simulink model "A7E_requirements"  (R2012b)
settings: Solver=ode45  StartTime=0.0  StopTime=10.0  RelTol=1e-3
libraries: sldvlib x4
settings Model: Creator=roberto  LastModifiedBy=roberto

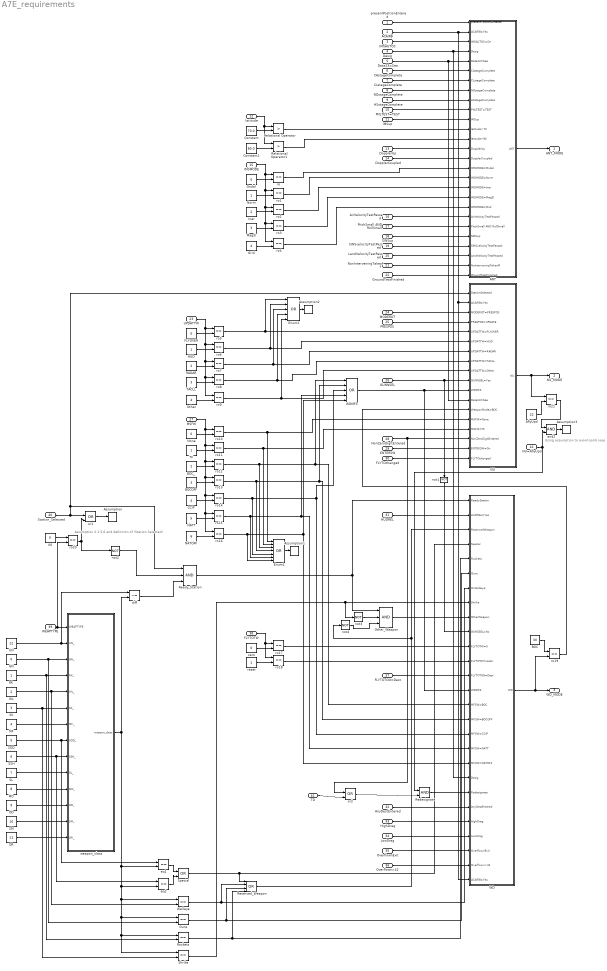
== system A7E_requirements ==
  note: Using assumption
      | to avoid comb loop
  note: Assumption 2.1.5.6
      | and definition
      | of !Station Selected!
  presentPositionEntered : Inport  OutDataTypeStr=boolean
  ACAIRB : Inport  Port=2  OutDataTypeStr=boolean
  IMSAUTOC : Inport  Port=3  OutDataTypeStr=boolean
  Desig : Inport  Port=4  OutDataTypeStr=boolean
  Data23=Sea : Inport  Port=5  OutDataTypeStr=boolean
  CAstageComplete : Inport  Port=6  OutDataTypeStr=boolean
  CLstageComplete : Inport  Port=7  OutDataTypeStr=boolean
  NDstageComplete : Inport  Port=8  OutDataTypeStr=boolean
  HSstageComplete : Inport  Port=9  OutDataTypeStr=boolean
  PNLTEST=TEST : Inport  Port=10  OutDataTypeStr=boolean
  IMSup : Inport  Port=11  OutDataTypeStr=boolean
  latitude : Inport  Port=12  OutDataTypeStr=double
  DopplerUp : Inport  Port=13  OutDataTypeStr=boolean
  DopplerCoupled : Inport  Port=14  OutDataTypeStr=boolean
  IMSMODE : Inport  Port=15  OutDataTypeStr=int8
  AirVelocityTestPassed : Inport  Port=16  OutDataTypeStr=boolean
  PitchSmall AND RollSmall : Inport  Port=17  OutDataTypeStr=boolean
  SINSup : Inport  Port=18  OutDataTypeStr=boolean
  SINSvelocityTestPassed : Inport  Port=19  OutDataTypeStr=boolean
  LandVelocityTestPassed : Inport  Port=20  OutDataTypeStr=boolean
  NonInterveningTakeoff : Inport  Port=21  OutDataTypeStr=boolean
  GroundTestFinished : Inport  Port=22  OutDataTypeStr=boolean
  UPDATTW : Inport  Port=23  OutDataTypeStr=int8
  MODEROT : Inport  Port=24  OutDataTypeStr=boolean
  PRESPOS : Inport  Port=25  OutDataTypeStr=boolean
  GUNNSEL : Inport  Port=26  OutDataTypeStr=boolean
  MSFW : Inport  Port=27  OutDataTypeStr=int8
  NonZeroDigitEntered : Inport  Port=28  OutDataTypeStr=boolean
  ENTERSW : Inport  Port=29  OutDataTypeStr=boolean
  FLYTOchanged : Inport  Port=30  OutDataTypeStr=boolean
  HUDREL : Inport  Port=31  OutDataTypeStr=boolean
  AnyDestEntered : Inport  Port=32  OutDataTypeStr=boolean
  HighDrag : Inport  Port=33  OutDataTypeStr=boolean
  LowDrag : Inport  Port=34  OutDataTypeStr=boolean
  OverflownExit : Inport  Port=35  OutDataTypeStr=boolean
  Overflown>42 : Inport  Port=36  OutDataTypeStr=boolean
  FLYTOTOG=Dest : Inport  Port=37  OutDataTypeStr=boolean
  FLYTOTW : Inport  Port=38  OutDataTypeStr=int8
  WEAPTYPE : Inport  Port=39  OutDataTypeStr=int8
  Station_Selected : Inport  Port=40  OutDataTypeStr=boolean
  TD : Inport  Port=41  OutDataTypeStr=boolean
  NU=AflyUpd : Inport  Port=42  OutDataTypeStr=boolean
  00 : Constant  Value=0  OutDataTypeStr=int8
  ANT : Subsystem
  AflyUpd : Constant  Value=22  OutDataTypeStr=int8
  Assumption{,1..3} (4 alike) : sldvlib/Objectives and Constraints/Assumption  enabled=on  customAVTBlockType=Assumption  intervals=true  initial=off  dispValues=on  outEnabled=on
      settings: AttributesFormatString=%<intervals>
  BOC : Constant  Value=30  OutDataTypeStr=int8
  BOCOFF : Constant  Value=3  OutDataTypeStr=int8
  BOC_ : Constant  Value=2  OutDataTypeStr=int8
  CCIP : Constant  Value=4  OutDataTypeStr=int8
  Constant : Constant  Value=70.0  OutDataTypeStr=double
  Constant1 : Constant  Value=80.0  OutDataTypeStr=double
  Enum1 : Logic  Operator=OR  Inputs=7  IconShape=distinctive  AllPortsSameDT=off  OutDataTypeStr=boolean
  Enum2 : Logic  Operator=OR  Inputs=5  IconShape=distinctive  AllPortsSameDT=off  OutDataTypeStr=boolean
  FLYOVER : Constant  Value=0  OutDataTypeStr=int8
  GN : Constant  Value=0  OutDataTypeStr=int8
  Gndal : Constant  Value=0  OutDataTypeStr=int8
  Grid : Constant  Value=4  OutDataTypeStr=int8
  Guns : RelationalOperator  Operator===  OutDataTypeStr=boolean
  HUD : Constant  OutDataTypeStr=int8
  Iner : Constant  Value=2  OutDataTypeStr=int8
  MD : Constant  Value=8  OutDataTypeStr=int8
  MF : Constant  Value=4  OutDataTypeStr=int8
  MagSl : Constant  Value=3  OutDataTypeStr=int8
  NATOFF : Constant  Value=6  OutDataTypeStr=int8
  NATT : Constant  Value=5  OutDataTypeStr=int8
  NU : Subsystem
  None : Constant  Value=0  OutDataTypeStr=int8
  Norm : Constant  OutDataTypeStr=int8
  OD : Constant  Value=9  OutDataTypeStr=int8
  OR : Constant  Value=11  OutDataTypeStr=int8
  Other : Constant  Value=4  OutDataTypeStr=int8
  Other_Weapon : Logic  Inputs=3  IconShape=distinctive  AllPortsSameDT=off  OutDataTypeStr=boolean
  RADAR : Constant  Value=2  OutDataTypeStr=int8
  RK : Constant  OutDataTypeStr=int8
  Ready_Station : Logic  Inputs=3  IconShape=distinctive  AllPortsSameDT=off  OutDataTypeStr=boolean
  Redesignate : Logic  IconShape=distinctive  AllPortsSameDT=off  OutDataTypeStr=boolean
  Relational Operator : RelationalOperator  Operator=>  OutDataTypeStr=boolean
  Relational Operator1 : RelationalOperator  Operator=>  OutDataTypeStr=boolean
  Reserved_Weapon : Logic  Operator=OR  Inputs=4  IconShape=distinctive  AllPortsSameDT=off  OutDataTypeStr=boolean
  Rockets : RelationalOperator  Operator===  OutDataTypeStr=boolean
  SK : Constant  Value=3  OutDataTypeStr=int8
  SL : Constant  Value=7  OutDataTypeStr=int8
  SM : Constant  Value=10  OutDataTypeStr=int8
  SOD : Constant  Value=5  OutDataTypeStr=int8
  SSH : Constant  Value=6  OutDataTypeStr=int8
  Shrike : RelationalOperator  Operator===  OutDataTypeStr=boolean
  Special : Logic  Operator=OR  IconShape=distinctive  AllPortsSameDT=off  OutDataTypeStr=boolean
  TACLL : Constant  Value=3  OutDataTypeStr=int8
  TF : Constant  OutDataTypeStr=int8
  UN : Constant  Value=12  OutDataTypeStr=int8
  WD : Subsystem
  WDMFS : Logic  Operator=OR  Inputs=5  IconShape=distinctive  AllPortsSameDT=off  OutDataTypeStr=boolean
  WL : Constant  Value=2  OutDataTypeStr=int8
  Walleye : RelationalOperator  Operator===  OutDataTypeStr=boolean
  and2 : Logic  IconShape=distinctive  AllPortsSameDT=off  OutDataTypeStr=boolean
  diff : RelationalOperator  Operator=~=  OutDataTypeStr=boolean
  eq1 : RelationalOperator  Operator===  OutDataTypeStr=boolean
  eq2 : RelationalOperator  Operator===  OutDataTypeStr=boolean
  not1 : Logic  Operator=NOT  IconShape=distinctive  AllPortsSameDT=off  OutDataTypeStr=boolean
  not2 : Logic  Operator=NOT  Inputs=3  IconShape=distinctive  AllPortsSameDT=off  OutDataTypeStr=boolean
  not3 : Logic  Operator=NOT  Inputs=3  IconShape=distinctive  AllPortsSameDT=off  OutDataTypeStr=boolean
  not4 : Logic  Operator=NOT  Inputs=3  IconShape=distinctive  AllPortsSameDT=off  OutDataTypeStr=boolean
  or1 : Logic  Operator=OR  IconShape=distinctive  AllPortsSameDT=off  OutDataTypeStr=boolean
  or2 : Logic  Operator=OR  IconShape=distinctive  AllPortsSameDT=off  OutDataTypeStr=boolean
  reset : Constant  OutDataTypeStr=int8
  ro{,1..21} (22 alike) : RelationalOperator  Operator===  OutDataTypeStr=boolean
  weapon_class : Subsystem
  zero : Constant  Value=0  OutDataTypeStr=int8
  ANT_MODE : Outport
  NU_MODE : Outport  Port=2
  WD_MODE : Outport  Port=3
  wires:
  presentPositionEntered/1 -> ANT/1(presentPositionEntered)
  ACAIRB/1 -> WD/27(ACAIRB=Yes), NU/2(ACAIRB=Yes), ANT/2(ACAIRB=Yes)
  IMSAUTOC/1 -> ANT/3(IMSAUTOC=On)
  Desig/1 -> WD/20(Desig), ANT/4(Desig)
  Data23=Sea/1 -> NU/12(Data23=Sea), ANT/5(Data23=Sea)
  CAstageComplete/1 -> ANT/6(CAstageComplete)
  CLstageComplete/1 -> ANT/7(CLstageComplete)
  NDstageComplete/1 -> ANT/8(NDstageComplete)
  HSstageComplete/1 -> ANT/9(HSstageComplete)
  PNLTEST=TEST/1 -> ANT/10(PNLTEST=TEST)
  IMSup/1 -> ANT/11(IMSup)
  DopplerUp/1 -> ANT/14(DopplerUp)
  DopplerCoupled/1 -> ANT/15(DopplerCoupled)
  AirVelocityTestPassed/1 -> ANT/21(AirVelocityTestPassed)
  PitchSmall AND RollSmall/1 -> ANT/22(PitchSmall AND RollSmall)
  ANT/1(ANT) -> ANT_MODE/1
  Station_Selected/1 -> NU/1(StationSelected), Ready_Station/1, or1/1
  latitude/1 -> Relational Operator1/1, Relational Operator/1
  Constant/1 -> Relational Operator/2
  Constant1/1 -> Relational Operator1/2
  Relational Operator1/1 -> ANT/13(latitude>80)
  Relational Operator/1 -> ANT/12(latitude>70)
  IMSMODE/1 -> ro/1, ro4/1, ro3/1, ro2/1, ro1/1
  Gndal/1 -> ro/2
  Norm/1 -> ro1/2
  Iner/1 -> ro2/2
  MagSl/1 -> ro3/2
  Grid/1 -> ro4/2
  ro/1 -> ANT/16(IMSMODE=Gndal)
  ro1/1 -> ANT/17(IMSMODE=Norm)
  ro2/1 -> ANT/18(IMSMODE=Iner)
  ro3/1 -> ANT/19(IMSMODE=MagSl)
  ro4/1 -> ANT/20(IMSMODE=Grid)
  UPDATTW/1 -> ro5/1, ro9/1, ro8/1, ro7/1, ro6/1
  FLYOVER/1 -> ro5/2
  HUD/1 -> ro6/2
  RADAR/1 -> ro7/2
  TACLL/1 -> ro8/2
  Other/1 -> ro9/2
  ro5/1 -> Enum2/1, NU/5(UPDATTW=FLYOVER)
  ro6/1 -> Enum2/2, NU/6(UPDATTW=HUD)
  ro7/1 -> Enum2/3, NU/7(UPDATTW=RADAR)
  ro8/1 -> Enum2/4, NU/8(UPDATTW=TACLL)
  ro9/1 -> Enum2/5, NU/9(UPDATTW=Other)
  MODEROT/1 -> NU/3(MODEROT=PRESPOS)
  PRESPOS/1 -> NU/4(PRESPOS=UPDATE)
  GUNNSEL/1 -> not1/1, NU/10(GUNNSEL=Yes)
  MSFW/1 -> ro10/1, ro16/1, ro15/1, ro14/1, ro13/1, ro12/1, ro11/1
  None/1 -> ro10/2
  TF/1 -> ro11/2
  BOC_/1 -> ro12/2
  BOCOFF/1 -> ro13/2
  CCIP/1 -> ro14/2
  NATT/1 -> ro15/2
  NATOFF/1 -> ro16/2
  ro10/1 -> Enum1/1, NU/14(MSFW=None)
  ro11/1 -> Enum1/2, NU/15(MSFW=TF)
  ro12/1 -> Enum1/3, WDMFS/1, WD/15(MFSW=BOC)
  ro13/1 -> Enum1/4, WDMFS/2, WD/16(MFSW=BOCOFF)
  ro14/1 -> Enum1/5, WD/17(MFSW=CCIP), WDMFS/3
  ro16/1 -> Enum1/7, WD/19(MFSW=NATOFF), WDMFS/5
  NonZeroDigitEntered/1 -> or2/1, NU/16(NonZeroDigitEntered)
  ENTERSW/1 -> NU/17(ENTERSW=On)
  FLYTOchanged/1 -> NU/18(FLYTOchanged)
  Ready_Station/1 -> WD/1(ReadyStation), Other_Weapon/1
  HUDREL/1 -> WD/2(HUDREL=Yes)
  Special/1 -> Reserved_Weapon/1, WD/4(Special)
  Walleye/1 -> Reserved_Weapon/2, WD/7(OnWalleye)
  Other_Weapon/1 -> WD/9(OtherWeapon)
  not1/1 -> WD/10(GUNSSEL=No)
  WDMFS/1 -> WD/14(WDMFS), NU/11(WDMFS)
  AnyDestEntered/1 -> WD/22(AnyDestEntered)
  HighDrag/1 -> WD/23(HighDrag)
  LowDrag/1 -> WD/24(LowDrag)
  OverflownExit/1 -> WD/25(OverflownExit)
  Overflown>42/1 -> WD/26(Overflown>42)
  FLYTOTOG=Dest/1 -> WD/13(FLYTOTOG=Dest)
  FLYTOTW/1 -> ro17/1, ro18/1
  zero/1 -> ro17/2
  reset/1 -> ro18/2
  ro17/1 -> WD/11(FLYTOTW=0)
  ro18/1 -> WD/12(FLYTOTW=reset)
  GroundTestFinished/1 -> ANT/27(GroundTestFinished)
  NonInterveningTakeoff/1 -> ANT/26(NoInterveningTakeoff)
  SINSup/1 -> ANT/23(SINSup)
  SINSvelocityTestPassed/1 -> ANT/24(SINSvelocityTestPassed)
  LandVelocityTestPassed/1 -> ANT/25(LandVelocityTestPassed)
  NU/1(NU) -> ro21/1, NU_MODE/1
  WD/1(WD) -> ro19/2, WD_MODE/1
  BOC/1 -> ro19/1
  ro19/1 -> NU/13(WeaponMode=BOC)
  WEAPTYPE/1 -> weapon_class/1(WEAPTYPE), ro20/2
  UN/1 -> diff/1, weapon_class/2(UN_)
  GN/1 -> Guns/2, weapon_class/3(GN_)
  RK/1 -> Rockets/2, weapon_class/4(RK_)
  SK/1 -> Shrike/2, weapon_class/6(SK_)
  MF/1 -> weapon_class/7(MF_)
  SOD/1 -> eq1/1, weapon_class/8(SOD_)
  SSH/1 -> eq2/1, weapon_class/9(SSH_)
  SL/1 -> weapon_class/10(SL_)
  MD/1 -> weapon_class/11(MD_)
  OD/1 -> weapon_class/12(OD_)
  SM/1 -> weapon_class/13(SM_)
  OR/1 -> weapon_class/14(OR_)
  00/1 -> ro20/1
  ro20/1 -> or1/2, not2/1
  or1/1 -> Assumption/1
  not2/1 -> Ready_Station/2
  diff/1 -> Ready_Station/3
  weapon_class/1(weapon_class) -> diff/2, Shrike/1, Rockets/1, Guns/1, Walleye/1, eq2/2, eq1/2
  eq1/1 -> Special/1
  eq2/1 -> Special/2
  WL/1 -> Walleye/2, weapon_class/5(WL_)
  Guns/1 -> Reserved_Weapon/3, WD/6(Guns)
  Rockets/1 -> Reserved_Weapon/4, WD/5(Rockets)
  Shrike/1 -> not3/1, WD/8(Shrike)
  Reserved_Weapon/1 -> WD/3(ReservedWeapon), not4/1
  not3/1 -> Other_Weapon/2
  not4/1 -> Other_Weapon/3
  ro15/1 -> Enum1/6, WDMFS/4, WD/18(MFSW=NATT)
  Enum1/1 -> Assumption1/1
  Enum2/1 -> Assumption2/1
  TD/1 -> or2/2
  or2/1 -> Redesignate/2
  Redesignate/1 -> WD/21(Redesignate)
  AflyUpd/1 -> ro21/2
  NU=AflyUpd/1 -> Redesignate/1, and2/2
  ro21/1 -> and2/1
  and2/1 -> Assumption3/1

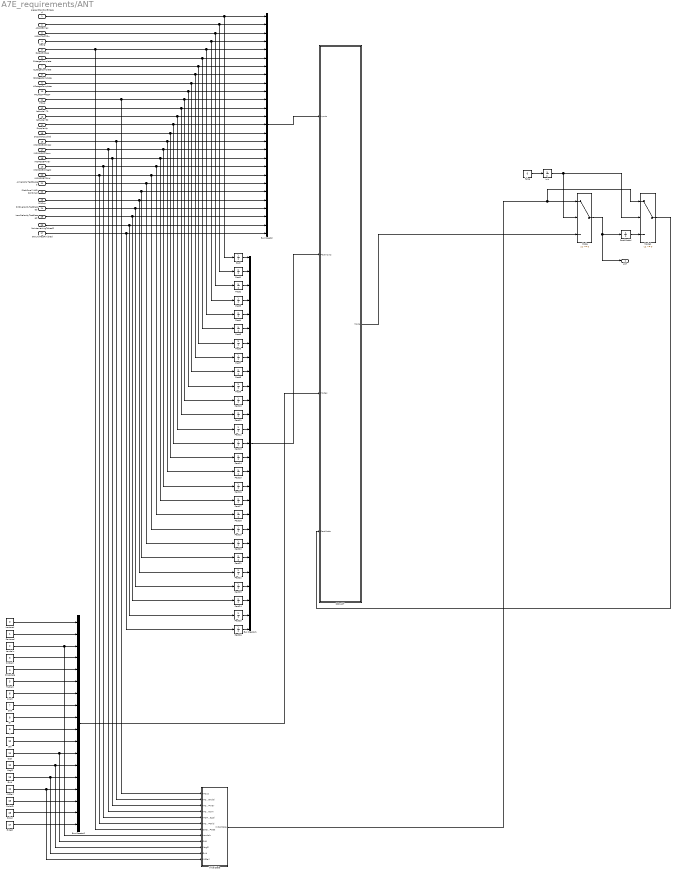
== system A7E_requirements/ANT ==
  presentPositionEntered : Inport  OutDataTypeStr=boolean
  ACAIRB=Yes : Inport  Port=2  OutDataTypeStr=boolean
  IMSAUTOC=On : Inport  Port=3  OutDataTypeStr=boolean
  Desig : Inport  Port=4  OutDataTypeStr=boolean
  Data23=Sea : Inport  Port=5  OutDataTypeStr=boolean
  CAstageComplete : Inport  Port=6  OutDataTypeStr=boolean
  CLstageComplete : Inport  Port=7  OutDataTypeStr=boolean
  NDstageComplete : Inport  Port=8  OutDataTypeStr=boolean
  HSstageComplete : Inport  Port=9  OutDataTypeStr=boolean
  PNLTEST=TEST : Inport  Port=10  OutDataTypeStr=boolean
  IMSup : Inport  Port=11  OutDataTypeStr=boolean
  latitude>70 : Inport  Port=12  OutDataTypeStr=boolean
  latitude>80 : Inport  Port=13  OutDataTypeStr=boolean
  DopplerUp : Inport  Port=14  OutDataTypeStr=boolean
  DopplerCoupled : Inport  Port=15  OutDataTypeStr=boolean
  IMSMODE=Gndal : Inport  Port=16  OutDataTypeStr=boolean
  IMSMODE=Norm : Inport  Port=17  OutDataTypeStr=boolean
  IMSMODE=Iner : Inport  Port=18  OutDataTypeStr=boolean
  IMSMODE=MagSl : Inport  Port=19  OutDataTypeStr=boolean
  IMSMODE=Grid : Inport  Port=20  OutDataTypeStr=boolean
  AirVelocityTestPassed : Inport  Port=21  OutDataTypeStr=boolean
  PitchSmall AND RollSmall : Inport  Port=22  OutDataTypeStr=boolean
  SINSup : Inport  Port=23  OutDataTypeStr=boolean
  SINSvelocityTestPassed : Inport  Port=24  OutDataTypeStr=boolean
  LandVelocityTestPassed : Inport  Port=25  OutDataTypeStr=boolean
  NoInterveningTakeoff : Inport  Port=26  OutDataTypeStr=boolean
  GroundTestFinished : Inport  Port=27  OutDataTypeStr=boolean
  01Update : Constant  Value=4  OutDataTypeStr=int8
  Airaln : Constant  Value=6  OutDataTypeStr=int8
  Bus Creator : BusCreator  Inputs=27
  Bus Creator1 : BusCreator  Inputs=27
  Bus Creator2 : BusCreator  Inputs=18
  DI : Constant  Value=8  OutDataTypeStr=int8
  DIG : Constant  Value=7  OutDataTypeStr=int8
  Grid : Constant  Value=13  OutDataTypeStr=int8
  Grtest : Constant  Value=17  OutDataTypeStr=int8
  HUDaln : Constant  Value=5  OutDataTypeStr=int8
  I : Constant  Value=9  OutDataTypeStr=int8
  IMSfail : Constant  Value=14  OutDataTypeStr=int8
  Init : UnitDelay  InitialCondition=1  SampleTime=-1
  InitialState : Subsystem
  Landaln : Constant  Value=2  OutDataTypeStr=int8
  Lautocal : Constant  Value=0  OutDataTypeStr=int8
  MagSl : Constant  Value=12  OutDataTypeStr=int8
  Mode : Switch  Criteria=u2 ~= 0  OutDataTypeStr=int8
  Mode1 : Switch  Criteria=u2 ~= 0  OutDataTypeStr=int8
  OLB : Constant  Value=11  OutDataTypeStr=int8
  Past{,1..26} (27 alike) : UnitDelay  InitialCondition=1  SampleTime=-1
  Past(Mode) : UnitDelay  InitialCondition=1  SampleTime=-1
  PolarDI : Constant  Value=15  OutDataTypeStr=int8
  PolarI : Constant  Value=16  OutDataTypeStr=int8
  SCR:ANT : Subsystem
  SINSaln : Constant  Value=3  OutDataTypeStr=int8
  Sautocal : Constant  OutDataTypeStr=int8
  UDI : Constant  Value=10  OutDataTypeStr=int8
  false : Constant  Value=0  OutDataTypeStr=boolean
  ANT : Outport
  wires:
  Past1/1 -> Bus Creator1/2
  Past4/1 -> Bus Creator1/5
  Past23/1 -> Bus Creator1/24
  Past20/1 -> Bus Creator1/21
  Past21/1 -> Bus Creator1/22
  Past6/1 -> Bus Creator1/7
  Past22/1 -> Bus Creator1/23
  Past5/1 -> Bus Creator1/6
  Past7/1 -> Bus Creator1/8
  Past24/1 -> Bus Creator1/25
  Past3/1 -> Bus Creator1/4
  Past2/1 -> Bus Creator1/3
  Past8/1 -> Bus Creator1/9
  Past9/1 -> Bus Creator1/10
  Past12/1 -> Bus Creator1/13
  Past11/1 -> Bus Creator1/12
  Past10/1 -> Bus Creator1/11
  Past17/1 -> Bus Creator1/18
  Past13/1 -> Bus Creator1/14
  Past14/1 -> Bus Creator1/15
  Past15/1 -> Bus Creator1/16
  Past18/1 -> Bus Creator1/19
  Past16/1 -> Bus Creator1/17
  Past19/1 -> Bus Creator1/20
  CLstageComplete/1 -> Past6/1, Bus Creator/7
  CAstageComplete/1 -> Past5/1, Bus Creator/6
  NDstageComplete/1 -> Past7/1, Bus Creator/8
  OLB/1 -> InitialState/9(OLB), Bus Creator2/12
  01Update/1 -> Bus Creator2/5
  HUDaln/1 -> Bus Creator2/6
  Airaln/1 -> Bus Creator2/7
  IMSfail/1 -> InitialState/12(IMSfail), Bus Creator2/15
  presentPositionEntered/1 -> Past/1, Bus Creator/1
  ACAIRB=Yes/1 -> Past1/1, Bus Creator/2
  PitchSmall AND RollSmall/1 -> Past21/1, Bus Creator/22
  SINSup/1 -> Past22/1, Bus Creator/23
  DopplerCoupled/1 -> Past14/1, Bus Creator/15
  PNLTEST=TEST/1 -> Past9/1, Bus Creator/10
  IMSMODE=Iner/1 -> InitialState/3(IMSMODE=Iner), Past17/1, Bus Creator/18
  IMSMODE=MagSl/1 -> InitialState/5(IMSMODE=MagSl), Past18/1, Bus Creator/19
  LandVelocityTestPassed/1 -> Past24/1, Bus Creator/25
  SINSvelocityTestPassed/1 -> Past23/1, Bus Creator/24
  latitude>80/1 -> Past12/1, Bus Creator/13
  IMSup/1 -> InitialState/1(IMSup), Past10/1, Bus Creator/11
  IMSMODE=Norm/1 -> InitialState/4(IMSMODE=Norm), Past16/1, Bus Creator/17
  AirVelocityTestPassed/1 -> Past20/1, Bus Creator/21
  IMSMODE=Grid/1 -> InitialState/6(IMSMODE=Grid), Past19/1, Bus Creator/20
  DopplerUp/1 -> Past13/1, Bus Creator/14
  HSstageComplete/1 -> Past8/1, Bus Creator/9
  IMSMODE=Gndal/1 -> InitialState/2(IMSMODE=Gndal), Past15/1, Bus Creator/16
  latitude>70/1 -> Past11/1, Bus Creator/12
  IMSAUTOC=On/1 -> Past2/1, Bus Creator/3
  Desig/1 -> Past3/1, Bus Creator/4
  Sautocal/1 -> Bus Creator2/2
  Landaln/1 -> Bus Creator2/3, InitialState/8(Landaln)
  SINSaln/1 -> Bus Creator2/4
  Past/1 -> Bus Creator1/1
  Mode/1 -> Past(Mode)/1, ANT/1
  Mode1/1 -> SCR:ANT/4(PastMode)
  SCR:ANT/1(Mode) -> Mode/3
  Bus Creator2/1 -> SCR:ANT/3(Modes)
  Bus Creator/1 -> SCR:ANT/1(Inputs)
  Bus Creator1/1 -> SCR:ANT/2(PastInputs)
  Init/1 -> Mode/2, Mode1/2
  Lautocal/1 -> Bus Creator2/1
  false/1 -> Init/1
  DI/1 -> Bus Creator2/9
  I/1 -> Bus Creator2/10
  DIG/1 -> Bus Creator2/8
  Grid/1 -> InitialState/11(Grid), Bus Creator2/14
  Grtest/1 -> Bus Creator2/18
  PolarI/1 -> Bus Creator2/17
  PolarDI/1 -> Bus Creator2/16
  UDI/1 -> Bus Creator2/11
  InitialState/1(InitialState) -> Mode1/1, Mode/1
  MagSl/1 -> InitialState/10(MagSl), Bus Creator2/13
  Data23=Sea/1 -> InitialState/7(Data23=Sea), Past4/1, Bus Creator/5
  NoInterveningTakeoff/1 -> Past25/1, Bus Creator/26
  GroundTestFinished/1 -> Past26/1, Bus Creator/27
  Past25/1 -> Bus Creator1/26
  Past26/1 -> Bus Creator1/27
  Past(Mode)/1 -> Mode1/3

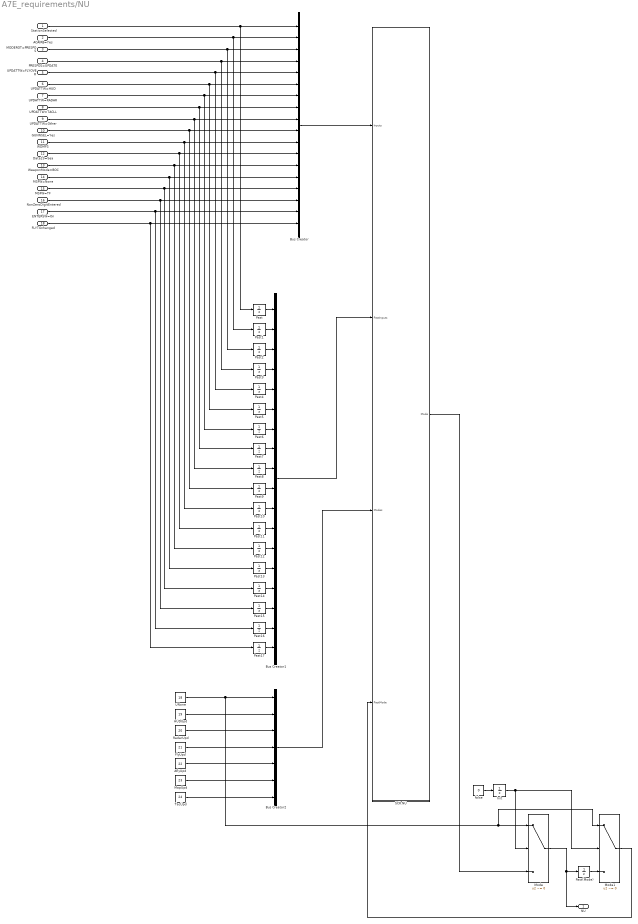
== system A7E_requirements/NU ==
  StationSelected : Inport  OutDataTypeStr=boolean
  ACAIRB=Yes : Inport  Port=2  OutDataTypeStr=boolean
  MODEROT=PRESPOS : Inport  Port=3  OutDataTypeStr=boolean
  PRESPOS=UPDATE : Inport  Port=4  OutDataTypeStr=boolean
  UPDATTW=FLYOVER : Inport  Port=5  OutDataTypeStr=boolean
  UPDATTW=HUD : Inport  Port=6  OutDataTypeStr=boolean
  UPDATTW=RADAR : Inport  Port=7  OutDataTypeStr=boolean
  UPDATTW=TACLL : Inport  Port=8  OutDataTypeStr=boolean
  UPDATTW=Other : Inport  Port=9  OutDataTypeStr=boolean
  GUNNSEL=Yes : Inport  Port=10  OutDataTypeStr=boolean
  WDMFS : Inport  Port=11  OutDataTypeStr=boolean
  Data23=Sea : Inport  Port=12  OutDataTypeStr=boolean
  WeaponMode=BOC : Inport  Port=13  OutDataTypeStr=boolean
  MSFW=None : Inport  Port=14  OutDataTypeStr=boolean
  MSFW=TF : Inport  Port=15  OutDataTypeStr=boolean
  NonZeroDigitEntered : Inport  Port=16  OutDataTypeStr=boolean
  ENTERSW=On : Inport  Port=17  OutDataTypeStr=boolean
  FLYTOchanged : Inport  Port=18  OutDataTypeStr=boolean
  AflyUpd : Constant  Value=22  OutDataTypeStr=int8
  Bus Creator : BusCreator  Inputs=18
  Bus Creator1 : BusCreator  Inputs=18
  Bus Creator2 : BusCreator  Inputs=7
  FlyUpd : Constant  Value=21  OutDataTypeStr=int8
  HUDUpd : Constant  Value=19  OutDataTypeStr=int8
  Init : UnitDelay  InitialCondition=1  SampleTime=-1
  MapUpd : Constant  Value=23  OutDataTypeStr=int8
  Mode : Switch  Criteria=u2 ~= 0
  Mode1 : Switch  Criteria=u2 ~= 0
  Past{,1..17} (18 alike) : UnitDelay  InitialCondition=1  SampleTime=-1
  Past(Mode) : UnitDelay  InitialCondition=1  SampleTime=-1
  RadarUpd : Constant  Value=20  OutDataTypeStr=int8
  SCR:NU : Subsystem
  TacUpd : Constant  Value=24  OutDataTypeStr=int8
  UNone : Constant  Value=18  OutDataTypeStr=int8
  false : Constant  Value=0  OutDataTypeStr=boolean
  NU : Outport  OutDataTypeStr=int8
  wires:
  Past1/1 -> Bus Creator1/2
  Past4/1 -> Bus Creator1/5
  Past6/1 -> Bus Creator1/7
  Past5/1 -> Bus Creator1/6
  Past7/1 -> Bus Creator1/8
  Past3/1 -> Bus Creator1/4
  Past2/1 -> Bus Creator1/3
  Past8/1 -> Bus Creator1/9
  Past9/1 -> Bus Creator1/10
  Past12/1 -> Bus Creator1/13
  Past11/1 -> Bus Creator1/12
  Past10/1 -> Bus Creator1/11
  Past17/1 -> Bus Creator1/18
  Past13/1 -> Bus Creator1/14
  Past14/1 -> Bus Creator1/15
  Past15/1 -> Bus Creator1/16
  Past16/1 -> Bus Creator1/17
  UPDATTW=RADAR/1 -> Past6/1, Bus Creator/7
  UPDATTW=HUD/1 -> Past5/1, Bus Creator/6
  UPDATTW=TACLL/1 -> Past7/1, Bus Creator/8
  UPDATTW=FLYOVER/1 -> Past4/1, Bus Creator/5
  StationSelected/1 -> Past/1, Bus Creator/1
  ACAIRB=Yes/1 -> Past1/1, Bus Creator/2
  MSFW=TF/1 -> Past14/1, Bus Creator/15
  GUNNSEL=Yes/1 -> Past9/1, Bus Creator/10
  FLYTOchanged/1 -> Past17/1, Bus Creator/18
  WeaponMode=BOC/1 -> Past12/1, Bus Creator/13
  WDMFS/1 -> Past10/1, Bus Creator/11
  ENTERSW=On/1 -> Past16/1, Bus Creator/17
  MSFW=None/1 -> Past13/1, Bus Creator/14
  UPDATTW=Other/1 -> Past8/1, Bus Creator/9
  NonZeroDigitEntered/1 -> Past15/1, Bus Creator/16
  Data23=Sea/1 -> Past11/1, Bus Creator/12
  MODEROT=PRESPOS/1 -> Past2/1, Bus Creator/3
  PRESPOS=UPDATE/1 -> Past3/1, Bus Creator/4
  Past/1 -> Bus Creator1/1
  Mode/1 -> Past(Mode)/1, NU/1
  Mode1/1 -> SCR:NU/4(PastMode)
  SCR:NU/1(Mode) -> Mode/3
  Bus Creator2/1 -> SCR:NU/3(Modes)
  Bus Creator/1 -> SCR:NU/1(Inputs)
  Bus Creator1/1 -> SCR:NU/2(PastInputs)
  Init/1 -> Mode/2, Mode1/2
  false/1 -> Init/1
  UNone/1 -> Mode1/1, Mode/1, Bus Creator2/1
  HUDUpd/1 -> Bus Creator2/2
  RadarUpd/1 -> Bus Creator2/3
  FlyUpd/1 -> Bus Creator2/4
  AflyUpd/1 -> Bus Creator2/5
  MapUpd/1 -> Bus Creator2/6
  TacUpd/1 -> Bus Creator2/7
  Past(Mode)/1 -> Mode1/3

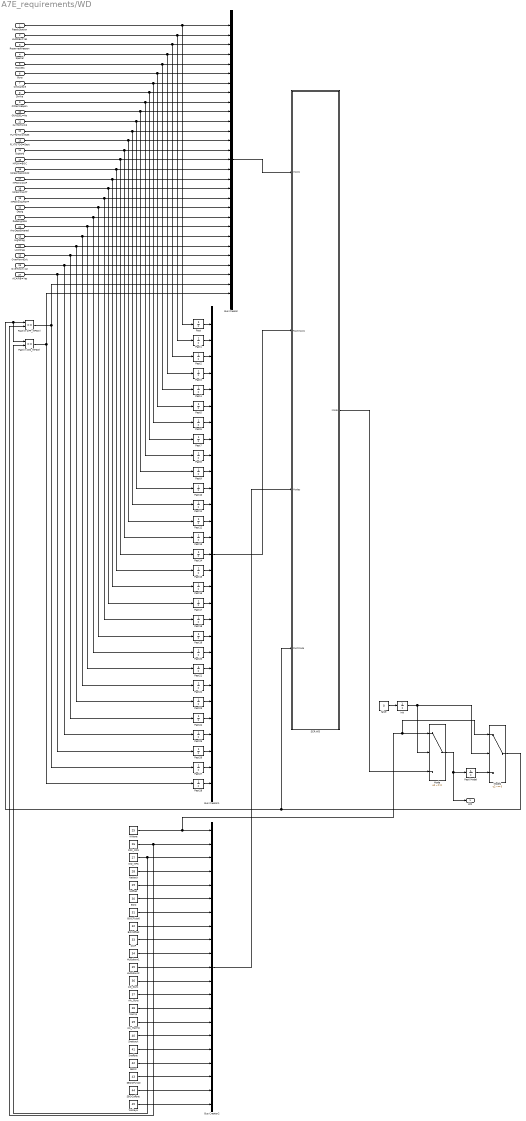
== system A7E_requirements/WD ==
  ReadyStation : Inport  OutDataTypeStr=boolean
  HUDREL=Yes : Inport  Port=2  OutDataTypeStr=boolean
  ReservedWeapon : Inport  Port=3  OutDataTypeStr=boolean
  Special : Inport  Port=4  OutDataTypeStr=boolean
  Rockets : Inport  Port=5  OutDataTypeStr=boolean
  Guns : Inport  Port=6  OutDataTypeStr=boolean
  OnWalleye : Inport  Port=7  OutDataTypeStr=boolean
  Shrike : Inport  Port=8  OutDataTypeStr=boolean
  OtherWeapon : Inport  Port=9  OutDataTypeStr=boolean
  GUNSSEL=No : Inport  Port=10  OutDataTypeStr=boolean
  FLYTOTW=0 : Inport  Port=11  OutDataTypeStr=boolean
  FLYTOTW=reset : Inport  Port=12  OutDataTypeStr=boolean
  FLYTOTOG=Dest : Inport  Port=13  OutDataTypeStr=boolean
  WDMFS : Inport  Port=14  OutDataTypeStr=boolean
  MFSW=BOC : Inport  Port=15  OutDataTypeStr=boolean
  MFSW=BOCOFF : Inport  Port=16  OutDataTypeStr=boolean
  MFSW=CCIP : Inport  Port=17  OutDataTypeStr=boolean
  MFSW=NATT : Inport  Port=18  OutDataTypeStr=boolean
  MFSW=NATOFF : Inport  Port=19  OutDataTypeStr=boolean
  Desig : Inport  Port=20  OutDataTypeStr=boolean
  Redesignate : Inport  Port=21  OutDataTypeStr=boolean
  AnyDestEntered : Inport  Port=22  OutDataTypeStr=boolean
  HighDrag : Inport  Port=23  OutDataTypeStr=boolean
  LowDrag : Inport  Port=24  OutDataTypeStr=boolean
  OverflownExit : Inport  Port=25  OutDataTypeStr=boolean
  Overflown>42 : Inport  Port=26  OutDataTypeStr=boolean
  ACAIRB=Yes : Inport  Port=27  OutDataTypeStr=boolean
  AA_Guns : Constant  Value=37  OutDataTypeStr=int8
  AA_Manrip : Constant  Value=39  OutDataTypeStr=int8
  AG_Guns : Constant  Value=36  OutDataTypeStr=int8
  BOC : Constant  Value=30  OutDataTypeStr=int8
  BOCFlyto0 : Constant  Value=31  OutDataTypeStr=int8
  BOCoffset : Constant  Value=32  OutDataTypeStr=int8
  Bus Creator : BusCreator  Inputs=29
  Bus Creator1 : BusCreator  Inputs=29
  Bus Creator2 : BusCreator  Inputs=21
  CCIP : Constant  Value=33  OutDataTypeStr=int8
  HUDdown1 : Constant  Value=34  OutDataTypeStr=int8
  HUDdown2 : Constant  Value=35  OutDataTypeStr=int8
  Init : UnitDelay  InitialCondition=1  SampleTime=-1
  Manrip : Constant  Value=38  OutDataTypeStr=int8
  Mode : Switch  Criteria=u2 ~= 0
  Mode1 : Switch  Criteria=u2 ~= 0
  Nattack : Constant  Value=28  OutDataTypeStr=int8
  Noffset : Constant  Value=29  OutDataTypeStr=int8
  OFF_MFS : Constant  Value=26  OutDataTypeStr=int8
  Past{,1..28} (29 alike) : UnitDelay  InitialCondition=1  SampleTime=-1
  Past(In OFF_MFSW) : RelationalOperator  Operator===  OutDataTypeStr=boolean
  Past(In WD_MFSW) : RelationalOperator  Operator===  OutDataTypeStr=boolean
  Past(Mode) : UnitDelay  InitialCondition=1  SampleTime=-1
  SBOC : Constant  Value=42  OutDataTypeStr=int8
  SBOCFlyto0 : Constant  Value=43  OutDataTypeStr=int8
  SBOCoffset : Constant  Value=44  OutDataTypeStr=int8
  SCR:WD : Subsystem
  Snattack : Constant  Value=40  OutDataTypeStr=int8
  Snoffset : Constant  Value=41  OutDataTypeStr=int8
  WD_MFS : Constant  Value=27  OutDataTypeStr=int8
  WNone : Constant  Value=25  OutDataTypeStr=int8
  Walleye : Constant  Value=45  OutDataTypeStr=int8
  false : Constant  Value=0  OutDataTypeStr=boolean
  WD : Outport
  wires:
  Past1/1 -> Bus Creator1/2
  Past4/1 -> Bus Creator1/5
  Past23/1 -> Bus Creator1/24
  Past20/1 -> Bus Creator1/21
  Past21/1 -> Bus Creator1/22
  Past6/1 -> Bus Creator1/7
  Past22/1 -> Bus Creator1/23
  Past5/1 -> Bus Creator1/6
  Past7/1 -> Bus Creator1/8
  Past24/1 -> Bus Creator1/25
  Past3/1 -> Bus Creator1/4
  Past2/1 -> Bus Creator1/3
  Past8/1 -> Bus Creator1/9
  Past9/1 -> Bus Creator1/10
  Past12/1 -> Bus Creator1/13
  Past11/1 -> Bus Creator1/12
  Past10/1 -> Bus Creator1/11
  Past17/1 -> Bus Creator1/18
  Past13/1 -> Bus Creator1/14
  Past14/1 -> Bus Creator1/15
  Past15/1 -> Bus Creator1/16
  Past18/1 -> Bus Creator1/19
  Past16/1 -> Bus Creator1/17
  Past19/1 -> Bus Creator1/20
  OnWalleye/1 -> Past6/1, Bus Creator/7
  Guns/1 -> Past5/1, Bus Creator/6
  Shrike/1 -> Past7/1, Bus Creator/8
  Rockets/1 -> Past4/1, Bus Creator/5
  AG_Guns/1 -> Bus Creator2/12
  BOC/1 -> Bus Creator2/6
  BOCFlyto0/1 -> Bus Creator2/7
  AA_Manrip/1 -> Bus Creator2/15
  ReadyStation/1 -> Past/1, Bus Creator/1
  HUDREL=Yes/1 -> Past1/1, Bus Creator/2
  AnyDestEntered/1 -> Past21/1, Bus Creator/22
  HighDrag/1 -> Past22/1, Bus Creator/23
  MFSW=BOC/1 -> Past14/1, Bus Creator/15
  GUNSSEL=No/1 -> Past9/1, Bus Creator/10
  MFSW=NATT/1 -> Past17/1, Bus Creator/18
  MFSW=NATOFF/1 -> Past18/1, Bus Creator/19
  OverflownExit/1 -> Past24/1, Bus Creator/25
  LowDrag/1 -> Past23/1, Bus Creator/24
  FLYTOTOG=Dest/1 -> Past12/1, Bus Creator/13
  FLYTOTW=0/1 -> Past10/1, Bus Creator/11
  MFSW=CCIP/1 -> Past16/1, Bus Creator/17
  Redesignate/1 -> Past20/1, Bus Creator/21
  Desig/1 -> Past19/1, Bus Creator/20
  WDMFS/1 -> Past13/1, Bus Creator/14
  OtherWeapon/1 -> Past8/1, Bus Creator/9
  MFSW=BOCOFF/1 -> Past15/1, Bus Creator/16
  FLYTOTW=reset/1 -> Past11/1, Bus Creator/12
  ReservedWeapon/1 -> Past2/1, Bus Creator/3
  Special/1 -> Past3/1, Bus Creator/4
  OFF_MFS/1 -> Past(In OFF_MFSW)/2, Bus Creator2/2
  WD_MFS/1 -> Past(In WD_MFSW)/2, Bus Creator2/3
  Nattack/1 -> Bus Creator2/4
  Past/1 -> Bus Creator1/1
  Mode/1 -> Past(Mode)/1, WD/1
  Mode1/1 -> Past(In WD_MFSW)/1, Past(In OFF_MFSW)/1, SCR:WD/4(PastMode)
  SCR:WD/1(Mode) -> Mode/3
  Bus Creator2/1 -> SCR:WD/3(Modes)
  Bus Creator/1 -> SCR:WD/1(Inputs)
  Bus Creator1/1 -> SCR:WD/2(PastInputs)
  Init/1 -> Mode/2, Mode1/2
  WNone/1 -> Mode1/1, Mode/1, Bus Creator2/1
  false/1 -> Init/1
  CCIP/1 -> Bus Creator2/9
  AA_Guns/1 -> Bus Creator2/13
  HUDdown1/1 -> Bus Creator2/10
  BOCoffset/1 -> Bus Creator2/8
  Manrip/1 -> Bus Creator2/14
  SBOC/1 -> Bus Creator2/18
  Snoffset/1 -> Bus Creator2/17
  Snattack/1 -> Bus Creator2/16
  HUDdown2/1 -> Bus Creator2/11
  Overflown>42/1 -> Past25/1, Bus Creator/26
  ACAIRB=Yes/1 -> Past26/1, Bus Creator/27
  Past(In OFF_MFSW)/1 -> Bus Creator/28, Past27/1
  Past(In WD_MFSW)/1 -> Bus Creator/29, Past28/1
  Past25/1 -> Bus Creator1/26
  Past26/1 -> Bus Creator1/27
  Past27/1 -> Bus Creator1/28
  Past28/1 -> Bus Creator1/29
  Noffset/1 -> Bus Creator2/5
  SBOCFlyto0/1 -> Bus Creator2/19
  SBOCoffset/1 -> Bus Creator2/20
  Walleye/1 -> Bus Creator2/21
  Past(Mode)/1 -> Mode1/3

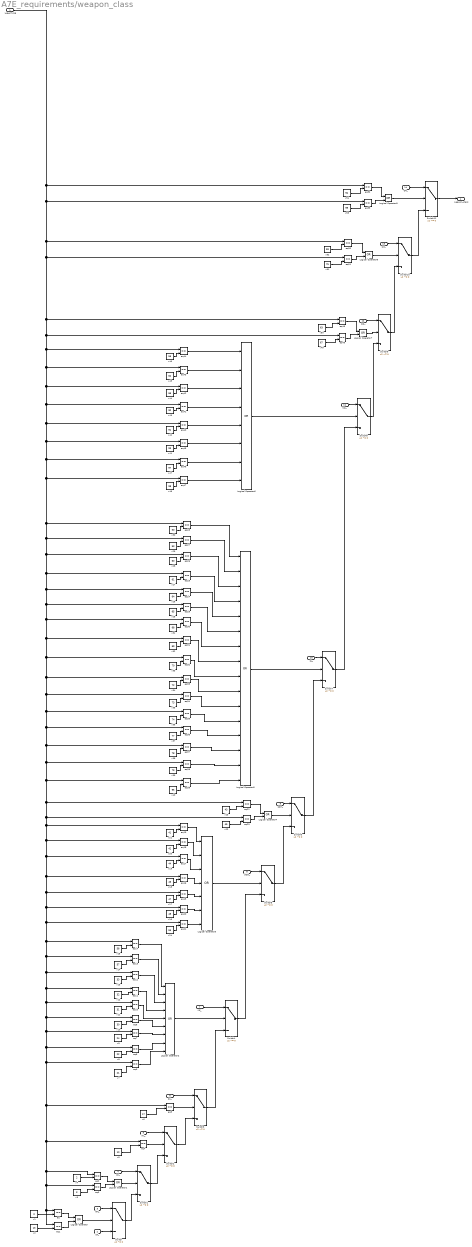
== system A7E_requirements/weapon_class ==
  WEAPTYPE : Inport  OutDataTypeStr=int8
  UN_ : Inport  Port=2  OutDataTypeStr=int8
  GN_ : Inport  Port=3  OutDataTypeStr=int8
  RK_ : Inport  Port=4  OutDataTypeStr=int8
  WL_ : Inport  Port=5  OutDataTypeStr=int8
  SK_ : Inport  Port=6  OutDataTypeStr=int8
  MF_ : Inport  Port=7  OutDataTypeStr=int8
  SOD_ : Inport  Port=8  OutDataTypeStr=int8
  SSH_ : Inport  Port=9  OutDataTypeStr=int8
  SL_ : Inport  Port=10  OutDataTypeStr=int8
  MD_ : Inport  Port=11  OutDataTypeStr=int8
  OD_ : Inport  Port=12  OutDataTypeStr=int8
  SM_ : Inport  Port=13  OutDataTypeStr=int8
  OR_ : Inport  Port=14  OutDataTypeStr=int8
  Logical Operator{,1,4,7..9} (6 alike) : Logic  Operator=OR  AllPortsSameDT=off  OutDataTypeStr=boolean
  Logical Operator2 : Logic  Operator=OR  Inputs=9  AllPortsSameDT=off  OutDataTypeStr=boolean
  Logical Operator3 : Logic  Operator=OR  Inputs=7  AllPortsSameDT=off  OutDataTypeStr=boolean
  Logical Operator5 : Logic  Operator=OR  Inputs=16  AllPortsSameDT=off  OutDataTypeStr=boolean
  Logical Operator6 : Logic  Operator=OR  Inputs=8  AllPortsSameDT=off  OutDataTypeStr=boolean
  Switch{,1..11} (12 alike) : Switch  Criteria=u2 ~= 0
  eq{,1..53} (54 alike) : RelationalOperator  Operator===  OutDataTypeStr=boolean
  v1 : Constant  Value=0  OutDataTypeStr=int8
  v10 : Constant  Value=30  OutDataTypeStr=int8
  v11 : Constant  Value=31  OutDataTypeStr=int8
  v12 : Constant  Value=32  OutDataTypeStr=int8
  v13 : Constant  Value=33  OutDataTypeStr=int8
  v14 : Constant  Value=57  OutDataTypeStr=int8
  v15 : Constant  Value=58  OutDataTypeStr=int8
  v16 : Constant  Value=48  OutDataTypeStr=int8
  v17 : Constant  Value=47  OutDataTypeStr=int8
  v18 : Constant  Value=46  OutDataTypeStr=int8
  v19 : Constant  Value=44  OutDataTypeStr=int8
  v2 : Constant  Value=13  OutDataTypeStr=int8
  v20 : Constant  Value=42  OutDataTypeStr=int8
  v21 : Constant  Value=41  OutDataTypeStr=int8
  v22 : Constant  Value=45  OutDataTypeStr=int8
  v23 : Constant  Value=43  OutDataTypeStr=int8
  v24 : Constant  Value=55  OutDataTypeStr=int8
  v25 : Constant  Value=65  OutDataTypeStr=int8
  v26 : Constant  Value=64  OutDataTypeStr=int8
  v27 : Constant  Value=61  OutDataTypeStr=int8
  v28 : Constant  Value=60  OutDataTypeStr=int8
  v29 : Constant  Value=53  OutDataTypeStr=int8
  v3 : Constant  Value=3  OutDataTypeStr=int8
  v30 : Constant  Value=50  OutDataTypeStr=int8
  v31 : Constant  Value=68  OutDataTypeStr=int8
  v32 : Constant  Value=69  OutDataTypeStr=int8
  v33 : Constant  Value=70  OutDataTypeStr=int8
  v34 : Constant  Value=72  OutDataTypeStr=int8
  v35 : Constant  Value=73  OutDataTypeStr=int8
  v36 : Constant  Value=74  OutDataTypeStr=int8
  v37 : Constant  Value=77  OutDataTypeStr=int8
  v38 : Constant  Value=78  OutDataTypeStr=int8
  v39 : Constant  Value=79  OutDataTypeStr=int8
  v4 : Constant  Value=2  OutDataTypeStr=int8
  v40 : Constant  Value=95  OutDataTypeStr=int8
  v41 : Constant  Value=93  OutDataTypeStr=int8
  v42 : Constant  Value=91  OutDataTypeStr=int8
  v43 : Constant  Value=90  OutDataTypeStr=int8
  v44 : Constant  Value=66  OutDataTypeStr=int8
  v45 : Constant  Value=62  OutDataTypeStr=int8
  v46 : Constant  Value=56  OutDataTypeStr=int8
  v47 : Constant  Value=97  OutDataTypeStr=int8
  v48 : Constant  Value=98  OutDataTypeStr=int8
  v49 : Constant  Value=67  OutDataTypeStr=int8
  v5 : Constant  Value=10  OutDataTypeStr=int8
  v50 : Constant  Value=63  OutDataTypeStr=int8
  v51 : Constant  Value=75  OutDataTypeStr=int8
  v52 : Constant  Value=59  OutDataTypeStr=int8
  v53 : Constant  Value=99  OutDataTypeStr=int8
  v54 : Constant  Value=94  OutDataTypeStr=int8
  v6 : Constant  Value=17  OutDataTypeStr=int8
  v7 : Constant  Value=21  OutDataTypeStr=int8
  v8 : Constant  Value=22  OutDataTypeStr=int8
  v9 : Constant  Value=24  OutDataTypeStr=int8
  weapon_class : Outport
  wires:
  v1/1 -> eq/2
  v2/1 -> eq1/2
  eq/1 -> Logical Operator/1
  eq1/1 -> Logical Operator/2
  Logical Operator/1 -> Switch/2
  GN_/1 -> Switch/1
  UN_/1 -> Switch/3
  Switch/1 -> Switch1/3
  Logical Operator1/1 -> Switch1/2
  eq3/1 -> Logical Operator1/2
  eq2/1 -> Logical Operator1/1
  v3/1 -> eq3/2
  v4/1 -> eq2/2
  Switch1/1 -> Switch2/3
  WL_/1 -> Switch2/1
  RK_/1 -> Switch1/1
  eq4/1 -> Switch2/2
  v5/1 -> eq4/2
  Switch2/1 -> Switch3/3
  SK_/1 -> Switch3/1
  eq5/1 -> Switch3/2
  v6/1 -> eq5/2
  Switch3/1 -> Switch4/3
  MF_/1 -> Switch4/1
  v7/1 -> eq9/2
  v8/1 -> eq8/2
  v9/1 -> eq7/2
  v10/1 -> eq6/2
  v11/1 -> eq10/2
  WEAPTYPE/1 -> eq48/1, eq49/1, eq47/1, eq27/1, eq26/1, eq25/1, eq29/1, eq30/1, eq32/1, eq34/1, eq35/1, eq36/1, eq37/1, eq38/1, eq39/1, eq22/1, eq18/1, eq17/1, eq16/1, eq15/1, eq20/1, eq21/1, eq14/1, eq13/1, eq11/1, eq8/1, eq9/1, eq5/1, eq4/1, eq2/1, eq3/1, eq1/1, eq/1, eq7/1, eq6/1, eq10/1, eq12/1, eq19/1, eq23/1, eq33/1, eq31/1, eq24/1, eq28/1, eq46/1, eq45/1, eq40/1, eq41/1, eq42/1, eq43/1, eq44/1, eq51/1, eq50/1, eq53/1, eq52/1
  v12/1 -> eq11/2
  v13/1 -> eq12/2
  v14/1 -> eq13/2
  v15/1 -> eq14/2
  Logical Operator2/1 -> Switch4/2
  eq14/1 -> Logical Operator2/1
  eq13/1 -> Logical Operator2/2
  eq12/1 -> Logical Operator2/3
  Switch4/1 -> Switch5/3
  SOD_/1 -> Switch5/1
  v24/1 -> eq21/2
  v16/1 -> eq20/2
  v17/1 -> eq15/2
  v18/1 -> eq16/2
  v19/1 -> eq17/2
  v20/1 -> eq18/2
  v21/1 -> eq19/2
  Logical Operator3/1 -> Switch5/2
  eq19/1 -> Logical Operator3/1
  eq18/1 -> Logical Operator3/2
  eq17/1 -> Logical Operator3/3
  eq11/1 -> Logical Operator2/4
  eq10/1 -> Logical Operator2/5
  eq6/1 -> Logical Operator2/6
  eq7/1 -> Logical Operator2/7
  eq8/1 -> Logical Operator2/8
  eq9/1 -> Logical Operator2/9
  eq21/1 -> Logical Operator3/7
  eq20/1 -> Logical Operator3/6
  eq15/1 -> Logical Operator3/5
  eq16/1 -> Logical Operator3/4
  SSH_/1 -> Switch6/1
  eq23/1 -> Logical Operator4/2
  eq22/1 -> Logical Operator4/1
  v22/1 -> eq23/2
  v23/1 -> eq22/2
  Logical Operator4/1 -> Switch6/2
  Switch5/1 -> Switch6/3
  SL_/1 -> Switch7/1
  Switch6/1 -> Switch7/3
  v31/1 -> eq30/2
  v25/1 -> eq29/2
  v26/1 -> eq24/2
  v27/1 -> eq25/2
  v28/1 -> eq26/2
  v29/1 -> eq27/2
  v30/1 -> eq28/2
  eq28/1 -> Logical Operator5/1
  eq27/1 -> Logical Operator5/2
  eq26/1 -> Logical Operator5/3
  eq30/1 -> Logical Operator5/7
  eq29/1 -> Logical Operator5/6
  eq24/1 -> Logical Operator5/5
  eq25/1 -> Logical Operator5/4
  v32/1 -> eq31/2
  eq31/1 -> Logical Operator5/8
  v33/1 -> eq32/2
  eq32/1 -> Logical Operator5/9
  v34/1 -> eq33/2
  eq33/1 -> Logical Operator5/10
  v35/1 -> eq34/2
  eq34/1 -> Logical Operator5/11
  v36/1 -> eq35/2
  eq35/1 -> Logical Operator5/12
  v37/1 -> eq36/2
  v38/1 -> eq37/2
  v39/1 -> eq38/2
  eq36/1 -> Logical Operator5/13
  eq37/1 -> Logical Operator5/14
  eq38/1 -> Logical Operator5/15
  v40/1 -> eq39/2
  eq39/1 -> Logical Operator5/16
  Logical Operator5/1 -> Switch7/2
  MD_/1 -> Switch8/1
  v47/1 -> eq46/2
  v41/1 -> eq45/2
  v42/1 -> eq40/2
  v43/1 -> eq41/2
  v44/1 -> eq42/2
  v45/1 -> eq43/2
  v46/1 -> eq44/2
  eq44/1 -> Logical Operator6/1
  eq43/1 -> Logical Operator6/2
  eq42/1 -> Logical Operator6/3
  eq46/1 -> Logical Operator6/7
  eq45/1 -> Logical Operator6/6
  eq40/1 -> Logical Operator6/5
  eq41/1 -> Logical Operator6/4
  v48/1 -> eq47/2
  eq47/1 -> Logical Operator6/8
  Logical Operator6/1 -> Switch8/2
  Switch7/1 -> Switch8/3
  OD_/1 -> Switch9/1
  eq49/1 -> Logical Operator7/2
  eq48/1 -> Logical Operator7/1
  v49/1 -> eq49/2
  v50/1 -> eq48/2
  Logical Operator7/1 -> Switch9/2
  Switch8/1 -> Switch9/3
  SM_/1 -> Switch10/1
  eq51/1 -> Logical Operator8/2
  eq50/1 -> Logical Operator8/1
  v51/1 -> eq51/2
  v52/1 -> eq50/2
  Logical Operator8/1 -> Switch10/2
  Switch9/1 -> Switch10/3
  Switch10/1 -> Switch11/3
  OR_/1 -> Switch11/1
  eq53/1 -> Logical Operator9/2
  eq52/1 -> Logical Operator9/1
  v53/1 -> eq53/2
  v54/1 -> eq52/2
  Logical Operator9/1 -> Switch11/2
  Switch11/1 -> weapon_class/1

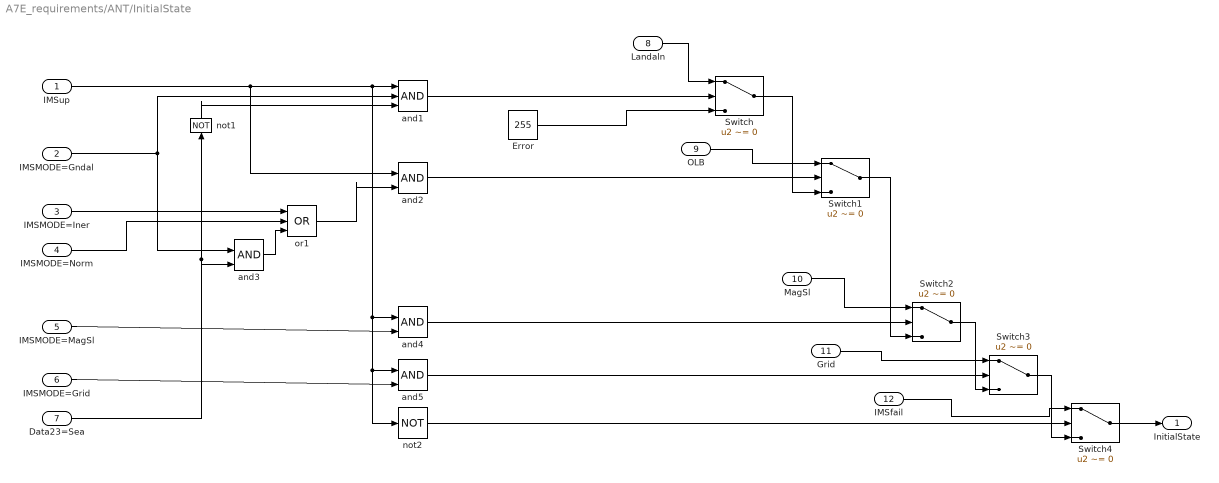
== system A7E_requirements/ANT/InitialState ==
  IMSup : Inport  OutDataTypeStr=boolean
  IMSMODE=Gndal : Inport  Port=2  OutDataTypeStr=boolean
  IMSMODE=Iner : Inport  Port=3  OutDataTypeStr=boolean
  IMSMODE=Norm : Inport  Port=4  OutDataTypeStr=boolean
  IMSMODE=MagSl : Inport  Port=5  OutDataTypeStr=boolean
  IMSMODE=Grid : Inport  Port=6  OutDataTypeStr=boolean
  Data23=Sea : Inport  Port=7  OutDataTypeStr=boolean
  Landaln : Inport  Port=8
  OLB : Inport  Port=9
  MagSl : Inport  Port=10
  Grid : Inport  Port=11
  IMSfail : Inport  Port=12
  Error : Constant  Value=255  OutDataTypeStr=int8
  Switch{,1..4} (5 alike) : Switch  Criteria=u2 ~= 0
  and1 : Logic  Inputs=3  IconShape=distinctive  AllPortsSameDT=off  OutDataTypeStr=boolean
  and{2..5} (4 alike) : Logic  IconShape=distinctive  AllPortsSameDT=off  OutDataTypeStr=boolean
  not1 : Logic  Operator=NOT  Inputs=3  IconShape=distinctive  AllPortsSameDT=off  OutDataTypeStr=boolean
  not2 : Logic  Operator=NOT  IconShape=distinctive  AllPortsSameDT=off  OutDataTypeStr=boolean
  or1 : Logic  Operator=OR  Inputs=3  IconShape=distinctive  AllPortsSameDT=off  OutDataTypeStr=boolean
  InitialState : Outport  OutDataTypeStr=int8
  wires:
  IMSup/1 -> and2/1, not2/1, and5/1, and4/1, and1/1
  IMSMODE=Gndal/1 -> and1/2, and3/1
  Data23=Sea/1 -> and3/2, not1/1
  not1/1 -> and1/3
  or1/1 -> and2/2
  and3/1 -> or1/3
  IMSMODE=Iner/1 -> or1/1
  IMSMODE=Norm/1 -> or1/2
  IMSMODE=MagSl/1 -> and4/2
  IMSMODE=Grid/1 -> and5/2
  and1/1 -> Switch/2
  Landaln/1 -> Switch/1
  Switch/1 -> Switch1/3
  and2/1 -> Switch1/2
  OLB/1 -> Switch1/1
  Switch1/1 -> Switch2/3
  MagSl/1 -> Switch2/1
  and4/1 -> Switch2/2
  and5/1 -> Switch3/2
  Switch2/1 -> Switch3/3
  Grid/1 -> Switch3/1
  not2/1 -> Switch4/2
  IMSfail/1 -> Switch4/1
  Switch4/1 -> InitialState/1
  Switch3/1 -> Switch4/3
  Error/1 -> Switch/3

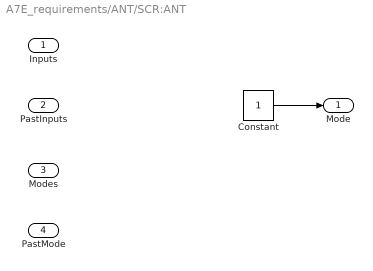
== system A7E_requirements/ANT/SCR:ANT ==
  Inputs : Inport
  PastInputs : Inport  Port=2
  Modes : Inport  Port=3
  PastMode : Inport  Port=4
  Constant : Constant  OutDataTypeStr=int8
  Mode : Outport  OutDataTypeStr=int8
  wires:
  Constant/1 -> Mode/1

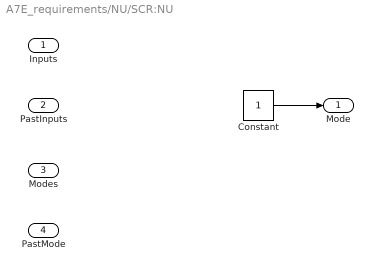
== system A7E_requirements/NU/SCR:NU ==
  Inputs : Inport
  PastInputs : Inport  Port=2
  Modes : Inport  Port=3
  PastMode : Inport  Port=4
  Constant : Constant  OutDataTypeStr=int8
  Mode : Outport
  wires:
  Constant/1 -> Mode/1

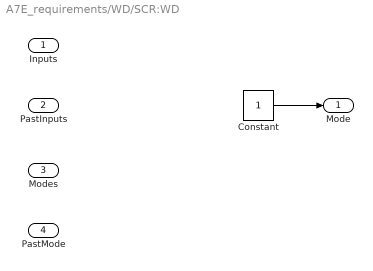
== system A7E_requirements/WD/SCR:WD ==
  Inputs : Inport
  PastInputs : Inport  Port=2
  Modes : Inport  Port=3
  PastMode : Inport  Port=4
  Constant : Constant  OutDataTypeStr=int8
  Mode : Outport
  wires:
  Constant/1 -> Mode/1
